simulink library "Kitchen_Lib"  (R2023a)
settings: Solver=VariableStepAuto  StartTime=0.0  StopTime=10.0  RelTol=1e-3  EnableMultiTasking=on
undefined symbols (not defined in the file): Kitc_BusTyp_P, Kitc_BusTypSkyr_C, Kitc_ColrLedColrls_C, Kitc_ColrLedGrn_C, Kitc_ColrLedRed_C, Kitc_ColrLedYlw_C, Kitc_StDgnWtrTank_C, Kitc_StElecPlugScktOffByClmp50_P, Kitc_StsDlyBlink_C, Kitc_StsErrBlink_C, Kitc_StsFctAcvn_P, Kitc_StsInfoBlink_C, Kitc_StsKitchnOffAutoIgOff_P, Kitc_StsKitchnOffBySwt_P, Kitc_StsKitchnOffDoorLockd_P, Kitc_StsKitchnOffIgOff_P, Kitc_StsKitchnOffUv_P, Kitc_StsKitchnOnBySwt_P, Kitc_StsKitchnOnNVM_P, Kitc_StsLedOff_C, Kitc_StsLedOn_C, Kitc_StsLrgCnsAcv_P, Kitc_StTrfrAnSwtInstd_P, Kitc_StTrfrSwtInstd_P, Kitc_TiKitcRefgtrOffDly_P, Kitc_ULowrThdBat_C, Kitc_UUpprThdBat_C, Kitc_ValFalse_C, Kitc_ValPwmFreq2_C, Kitc_ValPwmFreq_C, Kitc_ValTrue_C
libraries: MAN_Library x50, E2E_Lib x3
(part 12 of 13)

== system Kitchen_Lib/Kitchen/100ms/Kitchn/Subsystem1/Subsystem19/KSW_Battery/BatteryVoltageUnder23V/TurnOffDelay/TurnOffDelayOriginal/TimePulseOriginal/TimerCountingUpOriginal ==
  TimerEnable : Inport
  TimerReset : Inport  Port=2
  TimerThreshold : Inport  Port=3
  CycleTime : Inport  Port=4
  Data Type Conversion2 : DataTypeConversion  OutDataTypeStr=boolean  SaturateOnIntegerOverflow=off  RndMeth=Floor
  Data Type Conversion4 : DataTypeConversion  OutDataTypeStr=uint32  SaturateOnIntegerOverflow=off  RndMeth=Floor
  Data Type Conversion5 : DataTypeConversion  OutDataTypeStr=uint32  SaturateOnIntegerOverflow=off  RndMeth=Floor
  Data Type Conversion6 : DataTypeConversion  OutDataTypeStr=uint32  SaturateOnIntegerOverflow=off  RndMeth=Floor
  Data Type Conversion7 : DataTypeConversion  OutDataTypeStr=boolean  SaturateOnIntegerOverflow=off  RndMeth=Floor
  Delay : Delay  DelayLength=1  InitialCondition=0  ExternalReset=Rising
      settings: InputPortMap=u0,r5
  Delay1 : Delay  DelayLength=1  InitialCondition=0
  Logical Operator1 : Logic  Operator=NOT  AllPortsSameDT=off  OutDataTypeStr=boolean
  Logical Operator2 : Logic  AllPortsSameDT=off  OutDataTypeStr=boolean
  Logical Operator3 : Logic  Operator=OR  AllPortsSameDT=off  OutDataTypeStr=boolean
  Multiport Switch : MultiPortSwitch  DataPortOrder=Zero-based contiguous  Inputs=2  zeroidx=on  SaturateOnIntegerOverflow=off  InputSameDT=off
  Multiport Switch1 : MultiPortSwitch  DataPortOrder=Zero-based contiguous  Inputs=2  zeroidx=on  SaturateOnIntegerOverflow=off  InputSameDT=off
  Multiport Switch2 : MultiPortSwitch  DataPortOrder=Zero-based contiguous  Inputs=2  zeroidx=on  SaturateOnIntegerOverflow=off  InputSameDT=off
  Relational Operator : RelationalOperator  OutDataTypeStr=boolean  InputSameDT=off
  Relational Operator1 : RelationalOperator  Operator===  OutDataTypeStr=boolean  InputSameDT=off
  RisingEdgeDetection : Subsystem  AncestorBlock=MAN_Library/RisingEdgeDetection
  StartValue_ms1 : Constant  Value=uint32(4294967295)  OutDataTypeStr=uint32
  StartValue_ms2 : Constant  Value=uint32(4294967295)  OutDataTypeStr=uint32
  StartValue_ms3 : Constant  Value=uint32(0)  OutDataTypeStr=uint32
  StartValue_ms5 : Constant  Value=uint32(4294967295)  OutDataTypeStr=uint32
  Sum : Sum
  U32_Saturation : Subsystem  AncestorBlock=MAN_Library/U32_Saturation
  TimerFlag : Outport
  TimerCurrentValue : Outport  Port=2
  wires:
  CycleTime/1 -> Data Type Conversion4/1
  Data Type Conversion2/1 -> Logical Operator3/1
  RisingEdgeDetection/1(Q) -> Logical Operator3/2
  TimerReset/1 -> Data Type Conversion2/1
  TimerEnable/1 -> Data Type Conversion7/1
  Data Type Conversion6/1 -> Relational Operator/2
  Data Type Conversion4/1 -> Sum/2
  StartValue_ms3/1 -> U32_Saturation/3(LowerLimit), Multiport Switch/3
  Multiport Switch2/1 -> U32_Saturation/2(IN)
  Sum/1 -> Multiport Switch2/2
  StartValue_ms2/1 -> Multiport Switch2/3
  Relational Operator1/1 -> Multiport Switch2/1
  Delay/1 -> Multiport Switch1/2, Relational Operator1/1, Sum/1
  StartValue_ms5/1 -> Relational Operator1/2
  Logical Operator3/1 -> Multiport Switch/1, [ResetTimer_BOOL]
  StartValue_ms1/1 -> U32_Saturation/1(UpperLimit)
  Delay1/1 -> Logical Operator1/1
  U32_Saturation/1(OUT) -> Multiport Switch1/3
  Logical Operator1/1 -> Logical Operator2/2
  Logical Operator2/1 -> Multiport Switch1/1
  Data Type Conversion5/1 -> TimerCurrentValue/1, Delay/1, Relational Operator/1
  Data Type Conversion7/1 -> Logical Operator2/1, RisingEdgeDetection/1(CLK)
  Multiport Switch/1 -> Data Type Conversion5/1
  Relational Operator/1 -> TimerFlag/1, Delay1/1
  Multiport Switch1/1 -> Multiport Switch/2
  TimerThreshold/1 -> Data Type Conversion6/1
  [ResetTimer_BOOL] -> Delay/2

== system Kitchen_Lib/Kitchen/100ms/Kitchn/Subsystem1/Subsystem19/KitchenEnable/KitchenOffAutomaticIgnitionOff/TurnOnDelay/TurnOnDelayOriginal/TimePulseOriginal/RisingEdgeDetection ==
  CLK : Inport
  Constant : Constant  Value=boolean(1)  OutDataTypeStr=boolean
  Data Type Conversion1 : DataTypeConversion  OutDataTypeStr=boolean  SaturateOnIntegerOverflow=off  RndMeth=Floor
  Logical Operator : Logic  AllPortsSameDT=off  OutDataTypeStr=boolean
  Relational Operator : RelationalOperator  Operator=~=  OutDataTypeStr=boolean  InputSameDT=off
  Relational Operator1 : RelationalOperator  Operator===  OutDataTypeStr=boolean  InputSameDT=off
  Unit Delay : UnitDelay  SampleTime=-1  HasFrameUpgradeWarning=on
  Q : Outport
  wires:
  Data Type Conversion1/1 -> Relational Operator1/1, Relational Operator/2, Unit Delay/1
  Constant/1 -> Relational Operator1/2
  Logical Operator/1 -> Q/1
  Relational Operator1/1 -> Logical Operator/2
  Relational Operator/1 -> Logical Operator/1
  Unit Delay/1 -> Relational Operator/1
  CLK/1 -> Data Type Conversion1/1

== system Kitchen_Lib/Kitchen/100ms/Kitchn/Subsystem1/Subsystem19/KitchenEnable/KitchenOffAutomaticIgnitionOff/TurnOnDelay/TurnOnDelayOriginal/TimePulseOriginal/RisingEdgeDetection1 ==
  CLK : Inport
  Constant : Constant  Value=boolean(1)  OutDataTypeStr=boolean
  Data Type Conversion1 : DataTypeConversion  OutDataTypeStr=boolean  SaturateOnIntegerOverflow=off  RndMeth=Floor
  Logical Operator : Logic  AllPortsSameDT=off  OutDataTypeStr=boolean
  Relational Operator : RelationalOperator  Operator=~=  OutDataTypeStr=boolean  InputSameDT=off
  Relational Operator1 : RelationalOperator  Operator===  OutDataTypeStr=boolean  InputSameDT=off
  Unit Delay : UnitDelay  SampleTime=-1  HasFrameUpgradeWarning=on
  Q : Outport
  wires:
  Data Type Conversion1/1 -> Relational Operator1/1, Relational Operator/2, Unit Delay/1
  Constant/1 -> Relational Operator1/2
  Logical Operator/1 -> Q/1
  Relational Operator1/1 -> Logical Operator/2
  Relational Operator/1 -> Logical Operator/1
  Unit Delay/1 -> Relational Operator/1
  CLK/1 -> Data Type Conversion1/1

== system Kitchen_Lib/Kitchen/100ms/Kitchn/Subsystem1/Subsystem19/KitchenEnable/KitchenOffAutomaticIgnitionOff/TurnOnDelay/TurnOnDelayOriginal/TimePulseOriginal/SR ==
  S : Inport
  R : Inport  Port=2
  Constant1 : Constant  Value=boolean(1)  OutDataTypeStr=boolean
  Constant3 : Constant  Value=boolean(0)  OutDataTypeStr=boolean
  Data Type Conversion1 : DataTypeConversion  OutDataTypeStr=boolean  SaturateOnIntegerOverflow=off  RndMeth=Floor
  Data Type Conversion2 : DataTypeConversion  OutDataTypeStr=boolean  SaturateOnIntegerOverflow=off  RndMeth=Floor
  Multiport Switch : MultiPortSwitch  DataPortOrder=Zero-based contiguous  Inputs=2  zeroidx=on  SaturateOnIntegerOverflow=off  InputSameDT=off
  Multiport Switch1 : MultiPortSwitch  DataPortOrder=Zero-based contiguous  Inputs=2  zeroidx=on  SaturateOnIntegerOverflow=off  InputSameDT=off
  Unit Delay : UnitDelay  SampleTime=-1  HasFrameUpgradeWarning=on
  Q : Outport
  wires:
  Data Type Conversion2/1 -> Multiport Switch/1
  Data Type Conversion1/1 -> Multiport Switch1/1
  Constant3/1 -> Multiport Switch1/3
  Multiport Switch/1 -> Unit Delay/1, Q/1
  Unit Delay/1 -> Multiport Switch1/2
  R/1 -> Data Type Conversion1/1
  Multiport Switch1/1 -> Multiport Switch/2
  Constant1/1 -> Multiport Switch/3
  S/1 -> Data Type Conversion2/1

== system Kitchen_Lib/Kitchen/100ms/Kitchn/Subsystem1/Subsystem19/KitchenEnable/KitchenOffAutomaticIgnitionOff/TurnOnDelay/TurnOnDelayOriginal/TimePulseOriginal/TimerCountingUpOriginal ==
  TimerEnable : Inport
  TimerReset : Inport  Port=2
  TimerThreshold : Inport  Port=3
  CycleTime : Inport  Port=4
  Data Type Conversion2 : DataTypeConversion  OutDataTypeStr=boolean  SaturateOnIntegerOverflow=off  RndMeth=Floor
  Data Type Conversion4 : DataTypeConversion  OutDataTypeStr=uint32  SaturateOnIntegerOverflow=off  RndMeth=Floor
  Data Type Conversion5 : DataTypeConversion  OutDataTypeStr=uint32  SaturateOnIntegerOverflow=off  RndMeth=Floor
  Data Type Conversion6 : DataTypeConversion  OutDataTypeStr=uint32  SaturateOnIntegerOverflow=off  RndMeth=Floor
  Data Type Conversion7 : DataTypeConversion  OutDataTypeStr=boolean  SaturateOnIntegerOverflow=off  RndMeth=Floor
  Delay : Delay  DelayLength=1  InitialCondition=0  ExternalReset=Rising
      settings: InputPortMap=u0,r5
  Delay1 : Delay  DelayLength=1  InitialCondition=0
  Logical Operator1 : Logic  Operator=NOT  AllPortsSameDT=off  OutDataTypeStr=boolean
  Logical Operator2 : Logic  AllPortsSameDT=off  OutDataTypeStr=boolean
  Logical Operator3 : Logic  Operator=OR  AllPortsSameDT=off  OutDataTypeStr=boolean
  Multiport Switch : MultiPortSwitch  DataPortOrder=Zero-based contiguous  Inputs=2  zeroidx=on  SaturateOnIntegerOverflow=off  InputSameDT=off
  Multiport Switch1 : MultiPortSwitch  DataPortOrder=Zero-based contiguous  Inputs=2  zeroidx=on  SaturateOnIntegerOverflow=off  InputSameDT=off
  Multiport Switch2 : MultiPortSwitch  DataPortOrder=Zero-based contiguous  Inputs=2  zeroidx=on  SaturateOnIntegerOverflow=off  InputSameDT=off
  Relational Operator : RelationalOperator  OutDataTypeStr=boolean  InputSameDT=off
  Relational Operator1 : RelationalOperator  Operator===  OutDataTypeStr=boolean  InputSameDT=off
  RisingEdgeDetection : Subsystem  AncestorBlock=MAN_Library/RisingEdgeDetection
  StartValue_ms1 : Constant  Value=uint32(4294967295)  OutDataTypeStr=uint32
  StartValue_ms2 : Constant  Value=uint32(4294967295)  OutDataTypeStr=uint32
  StartValue_ms3 : Constant  Value=uint32(0)  OutDataTypeStr=uint32
  StartValue_ms5 : Constant  Value=uint32(4294967295)  OutDataTypeStr=uint32
  Sum : Sum
  U32_Saturation : Subsystem  AncestorBlock=MAN_Library/U32_Saturation
  TimerFlag : Outport
  TimerCurrentValue : Outport  Port=2
  wires:
  CycleTime/1 -> Data Type Conversion4/1
  Data Type Conversion2/1 -> Logical Operator3/1
  RisingEdgeDetection/1(Q) -> Logical Operator3/2
  TimerReset/1 -> Data Type Conversion2/1
  TimerEnable/1 -> Data Type Conversion7/1
  Data Type Conversion6/1 -> Relational Operator/2
  Data Type Conversion4/1 -> Sum/2
  StartValue_ms3/1 -> U32_Saturation/3(LowerLimit), Multiport Switch/3
  Multiport Switch2/1 -> U32_Saturation/2(IN)
  Sum/1 -> Multiport Switch2/2
  StartValue_ms2/1 -> Multiport Switch2/3
  Relational Operator1/1 -> Multiport Switch2/1
  Delay/1 -> Multiport Switch1/2, Relational Operator1/1, Sum/1
  StartValue_ms5/1 -> Relational Operator1/2
  Logical Operator3/1 -> Multiport Switch/1, [ResetTimer_BOOL]
  StartValue_ms1/1 -> U32_Saturation/1(UpperLimit)
  Delay1/1 -> Logical Operator1/1
  U32_Saturation/1(OUT) -> Multiport Switch1/3
  Logical Operator1/1 -> Logical Operator2/2
  Logical Operator2/1 -> Multiport Switch1/1
  Data Type Conversion5/1 -> TimerCurrentValue/1, Delay/1, Relational Operator/1
  Data Type Conversion7/1 -> Logical Operator2/1, RisingEdgeDetection/1(CLK)
  Multiport Switch/1 -> Data Type Conversion5/1
  Relational Operator/1 -> TimerFlag/1, Delay1/1
  Multiport Switch1/1 -> Multiport Switch/2
  TimerThreshold/1 -> Data Type Conversion6/1
  [ResetTimer_BOOL] -> Delay/2

== system Kitchen_Lib/Kitchen/100ms/Kitchn/Subsystem1/Subsystem19/KitchenEnable/Subsystem/TurnOnDelay/TurnOnDelayOriginal/TimePulseOriginal/RisingEdgeDetection ==
  CLK : Inport
  Constant : Constant  Value=boolean(1)  OutDataTypeStr=boolean
  Data Type Conversion1 : DataTypeConversion  OutDataTypeStr=boolean  SaturateOnIntegerOverflow=off  RndMeth=Floor
  Logical Operator : Logic  AllPortsSameDT=off  OutDataTypeStr=boolean
  Relational Operator : RelationalOperator  Operator=~=  OutDataTypeStr=boolean  InputSameDT=off
  Relational Operator1 : RelationalOperator  Operator===  OutDataTypeStr=boolean  InputSameDT=off
  Unit Delay : UnitDelay  SampleTime=-1  HasFrameUpgradeWarning=on
  Q : Outport
  wires:
  Data Type Conversion1/1 -> Relational Operator1/1, Relational Operator/2, Unit Delay/1
  Constant/1 -> Relational Operator1/2
  Logical Operator/1 -> Q/1
  Relational Operator1/1 -> Logical Operator/2
  Relational Operator/1 -> Logical Operator/1
  Unit Delay/1 -> Relational Operator/1
  CLK/1 -> Data Type Conversion1/1

== system Kitchen_Lib/Kitchen/100ms/Kitchn/Subsystem1/Subsystem19/KitchenEnable/Subsystem/TurnOnDelay/TurnOnDelayOriginal/TimePulseOriginal/RisingEdgeDetection1 ==
  CLK : Inport
  Constant : Constant  Value=boolean(1)  OutDataTypeStr=boolean
  Data Type Conversion1 : DataTypeConversion  OutDataTypeStr=boolean  SaturateOnIntegerOverflow=off  RndMeth=Floor
  Logical Operator : Logic  AllPortsSameDT=off  OutDataTypeStr=boolean
  Relational Operator : RelationalOperator  Operator=~=  OutDataTypeStr=boolean  InputSameDT=off
  Relational Operator1 : RelationalOperator  Operator===  OutDataTypeStr=boolean  InputSameDT=off
  Unit Delay : UnitDelay  SampleTime=-1  HasFrameUpgradeWarning=on
  Q : Outport
  wires:
  Data Type Conversion1/1 -> Relational Operator1/1, Relational Operator/2, Unit Delay/1
  Constant/1 -> Relational Operator1/2
  Logical Operator/1 -> Q/1
  Relational Operator1/1 -> Logical Operator/2
  Relational Operator/1 -> Logical Operator/1
  Unit Delay/1 -> Relational Operator/1
  CLK/1 -> Data Type Conversion1/1

== system Kitchen_Lib/Kitchen/100ms/Kitchn/Subsystem1/Subsystem19/KitchenEnable/Subsystem/TurnOnDelay/TurnOnDelayOriginal/TimePulseOriginal/SR ==
  S : Inport
  R : Inport  Port=2
  Constant1 : Constant  Value=boolean(1)  OutDataTypeStr=boolean
  Constant3 : Constant  Value=boolean(0)  OutDataTypeStr=boolean
  Data Type Conversion1 : DataTypeConversion  OutDataTypeStr=boolean  SaturateOnIntegerOverflow=off  RndMeth=Floor
  Data Type Conversion2 : DataTypeConversion  OutDataTypeStr=boolean  SaturateOnIntegerOverflow=off  RndMeth=Floor
  Multiport Switch : MultiPortSwitch  DataPortOrder=Zero-based contiguous  Inputs=2  zeroidx=on  SaturateOnIntegerOverflow=off  InputSameDT=off
  Multiport Switch1 : MultiPortSwitch  DataPortOrder=Zero-based contiguous  Inputs=2  zeroidx=on  SaturateOnIntegerOverflow=off  InputSameDT=off
  Unit Delay : UnitDelay  SampleTime=-1  HasFrameUpgradeWarning=on
  Q : Outport
  wires:
  Data Type Conversion2/1 -> Multiport Switch/1
  Data Type Conversion1/1 -> Multiport Switch1/1
  Constant3/1 -> Multiport Switch1/3
  Multiport Switch/1 -> Unit Delay/1, Q/1
  Unit Delay/1 -> Multiport Switch1/2
  R/1 -> Data Type Conversion1/1
  Multiport Switch1/1 -> Multiport Switch/2
  Constant1/1 -> Multiport Switch/3
  S/1 -> Data Type Conversion2/1

== system Kitchen_Lib/Kitchen/100ms/Kitchn/Subsystem1/Subsystem19/KitchenEnable/Subsystem/TurnOnDelay/TurnOnDelayOriginal/TimePulseOriginal/TimerCountingUpOriginal ==
  TimerEnable : Inport
  TimerReset : Inport  Port=2
  TimerThreshold : Inport  Port=3
  CycleTime : Inport  Port=4
  Data Type Conversion2 : DataTypeConversion  OutDataTypeStr=boolean  SaturateOnIntegerOverflow=off  RndMeth=Floor
  Data Type Conversion4 : DataTypeConversion  OutDataTypeStr=uint32  SaturateOnIntegerOverflow=off  RndMeth=Floor
  Data Type Conversion5 : DataTypeConversion  OutDataTypeStr=uint32  SaturateOnIntegerOverflow=off  RndMeth=Floor
  Data Type Conversion6 : DataTypeConversion  OutDataTypeStr=uint32  SaturateOnIntegerOverflow=off  RndMeth=Floor
  Data Type Conversion7 : DataTypeConversion  OutDataTypeStr=boolean  SaturateOnIntegerOverflow=off  RndMeth=Floor
  Delay : Delay  DelayLength=1  InitialCondition=0  ExternalReset=Rising
      settings: InputPortMap=u0,r5
  Delay1 : Delay  DelayLength=1  InitialCondition=0
  Logical Operator1 : Logic  Operator=NOT  AllPortsSameDT=off  OutDataTypeStr=boolean
  Logical Operator2 : Logic  AllPortsSameDT=off  OutDataTypeStr=boolean
  Logical Operator3 : Logic  Operator=OR  AllPortsSameDT=off  OutDataTypeStr=boolean
  Multiport Switch : MultiPortSwitch  DataPortOrder=Zero-based contiguous  Inputs=2  zeroidx=on  SaturateOnIntegerOverflow=off  InputSameDT=off
  Multiport Switch1 : MultiPortSwitch  DataPortOrder=Zero-based contiguous  Inputs=2  zeroidx=on  SaturateOnIntegerOverflow=off  InputSameDT=off
  Multiport Switch2 : MultiPortSwitch  DataPortOrder=Zero-based contiguous  Inputs=2  zeroidx=on  SaturateOnIntegerOverflow=off  InputSameDT=off
  Relational Operator : RelationalOperator  OutDataTypeStr=boolean  InputSameDT=off
  Relational Operator1 : RelationalOperator  Operator===  OutDataTypeStr=boolean  InputSameDT=off
  RisingEdgeDetection : Subsystem  AncestorBlock=MAN_Library/RisingEdgeDetection
  StartValue_ms1 : Constant  Value=uint32(4294967295)  OutDataTypeStr=uint32
  StartValue_ms2 : Constant  Value=uint32(4294967295)  OutDataTypeStr=uint32
  StartValue_ms3 : Constant  Value=uint32(0)  OutDataTypeStr=uint32
  StartValue_ms5 : Constant  Value=uint32(4294967295)  OutDataTypeStr=uint32
  Sum : Sum
  U32_Saturation : Subsystem  AncestorBlock=MAN_Library/U32_Saturation
  TimerFlag : Outport
  TimerCurrentValue : Outport  Port=2
  wires:
  CycleTime/1 -> Data Type Conversion4/1
  Data Type Conversion2/1 -> Logical Operator3/1
  RisingEdgeDetection/1(Q) -> Logical Operator3/2
  TimerReset/1 -> Data Type Conversion2/1
  TimerEnable/1 -> Data Type Conversion7/1
  Data Type Conversion6/1 -> Relational Operator/2
  Data Type Conversion4/1 -> Sum/2
  StartValue_ms3/1 -> U32_Saturation/3(LowerLimit), Multiport Switch/3
  Multiport Switch2/1 -> U32_Saturation/2(IN)
  Sum/1 -> Multiport Switch2/2
  StartValue_ms2/1 -> Multiport Switch2/3
  Relational Operator1/1 -> Multiport Switch2/1
  Delay/1 -> Multiport Switch1/2, Relational Operator1/1, Sum/1
  StartValue_ms5/1 -> Relational Operator1/2
  Logical Operator3/1 -> Multiport Switch/1, [ResetTimer_BOOL]
  StartValue_ms1/1 -> U32_Saturation/1(UpperLimit)
  Delay1/1 -> Logical Operator1/1
  U32_Saturation/1(OUT) -> Multiport Switch1/3
  Logical Operator1/1 -> Logical Operator2/2
  Logical Operator2/1 -> Multiport Switch1/1
  Data Type Conversion5/1 -> TimerCurrentValue/1, Delay/1, Relational Operator/1
  Data Type Conversion7/1 -> Logical Operator2/1, RisingEdgeDetection/1(CLK)
  Multiport Switch/1 -> Data Type Conversion5/1
  Relational Operator/1 -> TimerFlag/1, Delay1/1
  Multiport Switch1/1 -> Multiport Switch/2
  TimerThreshold/1 -> Data Type Conversion6/1
  [ResetTimer_BOOL] -> Delay/2

== system Kitchen_Lib/Kitchen/100ms/Kitchn/Subsystem1/Subsystem19/KitchenSwtLed/KitchenError/TurnOffDelay/TurnOffDelayOriginal/TimePulseOriginal/RisingEdgeDetection ==
  CLK : Inport
  Constant : Constant  Value=boolean(1)  OutDataTypeStr=boolean
  Data Type Conversion1 : DataTypeConversion  OutDataTypeStr=boolean  SaturateOnIntegerOverflow=off  RndMeth=Floor
  Logical Operator : Logic  AllPortsSameDT=off  OutDataTypeStr=boolean
  Relational Operator : RelationalOperator  Operator=~=  OutDataTypeStr=boolean  InputSameDT=off
  Relational Operator1 : RelationalOperator  Operator===  OutDataTypeStr=boolean  InputSameDT=off
  Unit Delay : UnitDelay  SampleTime=-1  HasFrameUpgradeWarning=on
  Q : Outport
  wires:
  Data Type Conversion1/1 -> Relational Operator1/1, Relational Operator/2, Unit Delay/1
  Constant/1 -> Relational Operator1/2
  Logical Operator/1 -> Q/1
  Relational Operator1/1 -> Logical Operator/2
  Relational Operator/1 -> Logical Operator/1
  Unit Delay/1 -> Relational Operator/1
  CLK/1 -> Data Type Conversion1/1

== system Kitchen_Lib/Kitchen/100ms/Kitchn/Subsystem1/Subsystem19/KitchenSwtLed/KitchenError/TurnOffDelay/TurnOffDelayOriginal/TimePulseOriginal/RisingEdgeDetection1 ==
  CLK : Inport
  Constant : Constant  Value=boolean(1)  OutDataTypeStr=boolean
  Data Type Conversion1 : DataTypeConversion  OutDataTypeStr=boolean  SaturateOnIntegerOverflow=off  RndMeth=Floor
  Logical Operator : Logic  AllPortsSameDT=off  OutDataTypeStr=boolean
  Relational Operator : RelationalOperator  Operator=~=  OutDataTypeStr=boolean  InputSameDT=off
  Relational Operator1 : RelationalOperator  Operator===  OutDataTypeStr=boolean  InputSameDT=off
  Unit Delay : UnitDelay  SampleTime=-1  HasFrameUpgradeWarning=on
  Q : Outport
  wires:
  Data Type Conversion1/1 -> Relational Operator1/1, Relational Operator/2, Unit Delay/1
  Constant/1 -> Relational Operator1/2
  Logical Operator/1 -> Q/1
  Relational Operator1/1 -> Logical Operator/2
  Relational Operator/1 -> Logical Operator/1
  Unit Delay/1 -> Relational Operator/1
  CLK/1 -> Data Type Conversion1/1

== system Kitchen_Lib/Kitchen/100ms/Kitchn/Subsystem1/Subsystem19/KitchenSwtLed/KitchenError/TurnOffDelay/TurnOffDelayOriginal/TimePulseOriginal/SR ==
  S : Inport
  R : Inport  Port=2
  Constant1 : Constant  Value=boolean(1)  OutDataTypeStr=boolean
  Constant3 : Constant  Value=boolean(0)  OutDataTypeStr=boolean
  Data Type Conversion1 : DataTypeConversion  OutDataTypeStr=boolean  SaturateOnIntegerOverflow=off  RndMeth=Floor
  Data Type Conversion2 : DataTypeConversion  OutDataTypeStr=boolean  SaturateOnIntegerOverflow=off  RndMeth=Floor
  Multiport Switch : MultiPortSwitch  DataPortOrder=Zero-based contiguous  Inputs=2  zeroidx=on  SaturateOnIntegerOverflow=off  InputSameDT=off
  Multiport Switch1 : MultiPortSwitch  DataPortOrder=Zero-based contiguous  Inputs=2  zeroidx=on  SaturateOnIntegerOverflow=off  InputSameDT=off
  Unit Delay : UnitDelay  SampleTime=-1  HasFrameUpgradeWarning=on
  Q : Outport
  wires:
  Data Type Conversion2/1 -> Multiport Switch/1
  Data Type Conversion1/1 -> Multiport Switch1/1
  Constant3/1 -> Multiport Switch1/3
  Multiport Switch/1 -> Unit Delay/1, Q/1
  Unit Delay/1 -> Multiport Switch1/2
  R/1 -> Data Type Conversion1/1
  Multiport Switch1/1 -> Multiport Switch/2
  Constant1/1 -> Multiport Switch/3
  S/1 -> Data Type Conversion2/1

== system Kitchen_Lib/Kitchen/100ms/Kitchn/Subsystem1/Subsystem19/KitchenSwtLed/KitchenError/TurnOffDelay/TurnOffDelayOriginal/TimePulseOriginal/TimerCountingUpOriginal ==
  TimerEnable : Inport
  TimerReset : Inport  Port=2
  TimerThreshold : Inport  Port=3
  CycleTime : Inport  Port=4
  Data Type Conversion2 : DataTypeConversion  OutDataTypeStr=boolean  SaturateOnIntegerOverflow=off  RndMeth=Floor
  Data Type Conversion4 : DataTypeConversion  OutDataTypeStr=uint32  SaturateOnIntegerOverflow=off  RndMeth=Floor
  Data Type Conversion5 : DataTypeConversion  OutDataTypeStr=uint32  SaturateOnIntegerOverflow=off  RndMeth=Floor
  Data Type Conversion6 : DataTypeConversion  OutDataTypeStr=uint32  SaturateOnIntegerOverflow=off  RndMeth=Floor
  Data Type Conversion7 : DataTypeConversion  OutDataTypeStr=boolean  SaturateOnIntegerOverflow=off  RndMeth=Floor
  Delay : Delay  DelayLength=1  InitialCondition=0  ExternalReset=Rising
      settings: InputPortMap=u0,r5
  Delay1 : Delay  DelayLength=1  InitialCondition=0
  Logical Operator1 : Logic  Operator=NOT  AllPortsSameDT=off  OutDataTypeStr=boolean
  Logical Operator2 : Logic  AllPortsSameDT=off  OutDataTypeStr=boolean
  Logical Operator3 : Logic  Operator=OR  AllPortsSameDT=off  OutDataTypeStr=boolean
  Multiport Switch : MultiPortSwitch  DataPortOrder=Zero-based contiguous  Inputs=2  zeroidx=on  SaturateOnIntegerOverflow=off  InputSameDT=off
  Multiport Switch1 : MultiPortSwitch  DataPortOrder=Zero-based contiguous  Inputs=2  zeroidx=on  SaturateOnIntegerOverflow=off  InputSameDT=off
  Multiport Switch2 : MultiPortSwitch  DataPortOrder=Zero-based contiguous  Inputs=2  zeroidx=on  SaturateOnIntegerOverflow=off  InputSameDT=off
  Relational Operator : RelationalOperator  OutDataTypeStr=boolean  InputSameDT=off
  Relational Operator1 : RelationalOperator  Operator===  OutDataTypeStr=boolean  InputSameDT=off
  RisingEdgeDetection : Subsystem  AncestorBlock=MAN_Library/RisingEdgeDetection
  StartValue_ms1 : Constant  Value=uint32(4294967295)  OutDataTypeStr=uint32
  StartValue_ms2 : Constant  Value=uint32(4294967295)  OutDataTypeStr=uint32
  StartValue_ms3 : Constant  Value=uint32(0)  OutDataTypeStr=uint32
  StartValue_ms5 : Constant  Value=uint32(4294967295)  OutDataTypeStr=uint32
  Sum : Sum
  U32_Saturation : Subsystem  AncestorBlock=MAN_Library/U32_Saturation
  TimerFlag : Outport
  TimerCurrentValue : Outport  Port=2
  wires:
  CycleTime/1 -> Data Type Conversion4/1
  Data Type Conversion2/1 -> Logical Operator3/1
  RisingEdgeDetection/1(Q) -> Logical Operator3/2
  TimerReset/1 -> Data Type Conversion2/1
  TimerEnable/1 -> Data Type Conversion7/1
  Data Type Conversion6/1 -> Relational Operator/2
  Data Type Conversion4/1 -> Sum/2
  StartValue_ms3/1 -> U32_Saturation/3(LowerLimit), Multiport Switch/3
  Multiport Switch2/1 -> U32_Saturation/2(IN)
  Sum/1 -> Multiport Switch2/2
  StartValue_ms2/1 -> Multiport Switch2/3
  Relational Operator1/1 -> Multiport Switch2/1
  Delay/1 -> Multiport Switch1/2, Relational Operator1/1, Sum/1
  StartValue_ms5/1 -> Relational Operator1/2
  Logical Operator3/1 -> Multiport Switch/1, [ResetTimer_BOOL]
  StartValue_ms1/1 -> U32_Saturation/1(UpperLimit)
  Delay1/1 -> Logical Operator1/1
  U32_Saturation/1(OUT) -> Multiport Switch1/3
  Logical Operator1/1 -> Logical Operator2/2
  Logical Operator2/1 -> Multiport Switch1/1
  Data Type Conversion5/1 -> TimerCurrentValue/1, Delay/1, Relational Operator/1
  Data Type Conversion7/1 -> Logical Operator2/1, RisingEdgeDetection/1(CLK)
  Multiport Switch/1 -> Data Type Conversion5/1
  Relational Operator/1 -> TimerFlag/1, Delay1/1
  Multiport Switch1/1 -> Multiport Switch/2
  TimerThreshold/1 -> Data Type Conversion6/1
  [ResetTimer_BOOL] -> Delay/2

== system Kitchen_Lib/Kitchen/100ms/Kitchn/Subsystem1/Subsystem19/KitchenSwtLed/TurnOffDelay1/TurnOffDelayOriginal/TimePulseOriginal/TimerCountingUpOriginal/RisingEdgeDetection ==
  CLK : Inport
  Constant : Constant  Value=boolean(1)  OutDataTypeStr=boolean
  Data Type Conversion1 : DataTypeConversion  OutDataTypeStr=boolean  SaturateOnIntegerOverflow=off  RndMeth=Floor
  Logical Operator : Logic  AllPortsSameDT=off  OutDataTypeStr=boolean
  Relational Operator : RelationalOperator  Operator=~=  OutDataTypeStr=boolean  InputSameDT=off
  Relational Operator1 : RelationalOperator  Operator===  OutDataTypeStr=boolean  InputSameDT=off
  Unit Delay : UnitDelay  SampleTime=-1  HasFrameUpgradeWarning=on
  Q : Outport
  wires:
  Data Type Conversion1/1 -> Relational Operator1/1, Relational Operator/2, Unit Delay/1
  Constant/1 -> Relational Operator1/2
  Logical Operator/1 -> Q/1
  Relational Operator1/1 -> Logical Operator/2
  Relational Operator/1 -> Logical Operator/1
  Unit Delay/1 -> Relational Operator/1
  CLK/1 -> Data Type Conversion1/1

== system Kitchen_Lib/Kitchen/100ms/Kitchn/Subsystem1/Subsystem19/KitchenSwtLed/TurnOffDelay1/TurnOffDelayOriginal/TimePulseOriginal/TimerCountingUpOriginal/U32_Saturation ==
  UpperLimit : Inport
  IN : Inport  Port=2
  LowerLimit : Inport  Port=3
  Data Type Conversion{1..4} (4 alike) : DataTypeConversion  OutDataTypeStr=uint32  SaturateOnIntegerOverflow=off  RndMeth=Floor
  MinMax : MinMax  Inputs=2  OutDataTypeStr=uint32
  MinMax1 : MinMax  Function=max  Inputs=2  OutDataTypeStr=uint32
  OUT : Outport
  wires:
  Data Type Conversion3/1 -> OUT/1
  Data Type Conversion2/1 -> MinMax/1
  Data Type Conversion1/1 -> MinMax/2
  Data Type Conversion4/1 -> MinMax1/1
  MinMax1/1 -> Data Type Conversion3/1
  LowerLimit/1 -> Data Type Conversion4/1
  MinMax/1 -> MinMax1/2
  IN/1 -> Data Type Conversion2/1
  UpperLimit/1 -> Data Type Conversion1/1

== system Kitchen_Lib/Kitchen/100ms/Kitchn/Subsystem1/Subsystem19/Refgtr/TurnOffDelay/TurnOffDelayOriginal/TimePulseOriginal/TimerCountingUpOriginal/RisingEdgeDetection ==
  CLK : Inport
  Constant : Constant  Value=boolean(1)  OutDataTypeStr=boolean
  Data Type Conversion1 : DataTypeConversion  OutDataTypeStr=boolean  SaturateOnIntegerOverflow=off  RndMeth=Floor
  Logical Operator : Logic  AllPortsSameDT=off  OutDataTypeStr=boolean
  Relational Operator : RelationalOperator  Operator=~=  OutDataTypeStr=boolean  InputSameDT=off
  Relational Operator1 : RelationalOperator  Operator===  OutDataTypeStr=boolean  InputSameDT=off
  Unit Delay : UnitDelay  SampleTime=-1  HasFrameUpgradeWarning=on
  Q : Outport
  wires:
  Data Type Conversion1/1 -> Relational Operator1/1, Relational Operator/2, Unit Delay/1
  Constant/1 -> Relational Operator1/2
  Logical Operator/1 -> Q/1
  Relational Operator1/1 -> Logical Operator/2
  Relational Operator/1 -> Logical Operator/1
  Unit Delay/1 -> Relational Operator/1
  CLK/1 -> Data Type Conversion1/1

== system Kitchen_Lib/Kitchen/100ms/Kitchn/Subsystem1/Subsystem19/Refgtr/TurnOffDelay/TurnOffDelayOriginal/TimePulseOriginal/TimerCountingUpOriginal/U32_Saturation ==
  UpperLimit : Inport
  IN : Inport  Port=2
  LowerLimit : Inport  Port=3
  Data Type Conversion{1..4} (4 alike) : DataTypeConversion  OutDataTypeStr=uint32  SaturateOnIntegerOverflow=off  RndMeth=Floor
  MinMax : MinMax  Inputs=2  OutDataTypeStr=uint32
  MinMax1 : MinMax  Function=max  Inputs=2  OutDataTypeStr=uint32
  OUT : Outport
  wires:
  Data Type Conversion3/1 -> OUT/1
  Data Type Conversion2/1 -> MinMax/1
  Data Type Conversion1/1 -> MinMax/2
  Data Type Conversion4/1 -> MinMax1/1
  MinMax1/1 -> Data Type Conversion3/1
  LowerLimit/1 -> Data Type Conversion4/1
  MinMax/1 -> MinMax1/2
  IN/1 -> Data Type Conversion2/1
  UpperLimit/1 -> Data Type Conversion1/1

== system Kitchen_Lib/Kitchen/100ms/Kitchn/Subsystem1/Subsystem19/Trfr/TurnOnDelay/TurnOnDelayOriginal/TimePulseOriginal/TimerCountingUpOriginal/RisingEdgeDetection ==
  CLK : Inport
  Constant : Constant  Value=boolean(1)  OutDataTypeStr=boolean
  Data Type Conversion1 : DataTypeConversion  OutDataTypeStr=boolean  SaturateOnIntegerOverflow=off  RndMeth=Floor
  Logical Operator : Logic  AllPortsSameDT=off  OutDataTypeStr=boolean
  Relational Operator : RelationalOperator  Operator=~=  OutDataTypeStr=boolean  InputSameDT=off
  Relational Operator1 : RelationalOperator  Operator===  OutDataTypeStr=boolean  InputSameDT=off
  Unit Delay : UnitDelay  SampleTime=-1  HasFrameUpgradeWarning=on
  Q : Outport
  wires:
  Data Type Conversion1/1 -> Relational Operator1/1, Relational Operator/2, Unit Delay/1
  Constant/1 -> Relational Operator1/2
  Logical Operator/1 -> Q/1
  Relational Operator1/1 -> Logical Operator/2
  Relational Operator/1 -> Logical Operator/1
  Unit Delay/1 -> Relational Operator/1
  CLK/1 -> Data Type Conversion1/1

== system Kitchen_Lib/Kitchen/100ms/Kitchn/Subsystem1/Subsystem19/Trfr/TurnOnDelay/TurnOnDelayOriginal/TimePulseOriginal/TimerCountingUpOriginal/U32_Saturation ==
  UpperLimit : Inport
  IN : Inport  Port=2
  LowerLimit : Inport  Port=3
  Data Type Conversion{1..4} (4 alike) : DataTypeConversion  OutDataTypeStr=uint32  SaturateOnIntegerOverflow=off  RndMeth=Floor
  MinMax : MinMax  Inputs=2  OutDataTypeStr=uint32
  MinMax1 : MinMax  Function=max  Inputs=2  OutDataTypeStr=uint32
  OUT : Outport
  wires:
  Data Type Conversion3/1 -> OUT/1
  Data Type Conversion2/1 -> MinMax/1
  Data Type Conversion1/1 -> MinMax/2
  Data Type Conversion4/1 -> MinMax1/1
  MinMax1/1 -> Data Type Conversion3/1
  LowerLimit/1 -> Data Type Conversion4/1
  MinMax/1 -> MinMax1/2
  IN/1 -> Data Type Conversion2/1
  UpperLimit/1 -> Data Type Conversion1/1

== system Kitchen_Lib/Kitchen/100ms/Kitchn/Subsystem1/Subsystem19/WaterTankEmptyDiagnostic/Diagno sticsDebouncing/DiagnosticsDebouncingOriginal/TurnOffDelayOriginal /TimePulseOriginal/RisingEdgeDetection ==
  CLK : Inport
  Constant : Constant  Value=boolean(1)  OutDataTypeStr=boolean
  Data Type Conversion1 : DataTypeConversion  OutDataTypeStr=boolean  SaturateOnIntegerOverflow=off  RndMeth=Floor
  Logical Operator : Logic  AllPortsSameDT=off  OutDataTypeStr=boolean
  Relational Operator : RelationalOperator  Operator=~=  OutDataTypeStr=boolean  InputSameDT=off
  Relational Operator1 : RelationalOperator  Operator===  OutDataTypeStr=boolean  InputSameDT=off
  Unit Delay : UnitDelay  SampleTime=-1  HasFrameUpgradeWarning=on
  Q : Outport
  wires:
  Data Type Conversion1/1 -> Relational Operator1/1, Relational Operator/2, Unit Delay/1
  Constant/1 -> Relational Operator1/2
  Logical Operator/1 -> Q/1
  Relational Operator1/1 -> Logical Operator/2
  Relational Operator/1 -> Logical Operator/1
  Unit Delay/1 -> Relational Operator/1
  CLK/1 -> Data Type Conversion1/1

== system Kitchen_Lib/Kitchen/100ms/Kitchn/Subsystem1/Subsystem19/WaterTankEmptyDiagnostic/Diagno sticsDebouncing/DiagnosticsDebouncingOriginal/TurnOffDelayOriginal /TimePulseOriginal/RisingEdgeDetection1 ==
  CLK : Inport
  Constant : Constant  Value=boolean(1)  OutDataTypeStr=boolean
  Data Type Conversion1 : DataTypeConversion  OutDataTypeStr=boolean  SaturateOnIntegerOverflow=off  RndMeth=Floor
  Logical Operator : Logic  AllPortsSameDT=off  OutDataTypeStr=boolean
  Relational Operator : RelationalOperator  Operator=~=  OutDataTypeStr=boolean  InputSameDT=off
  Relational Operator1 : RelationalOperator  Operator===  OutDataTypeStr=boolean  InputSameDT=off
  Unit Delay : UnitDelay  SampleTime=-1  HasFrameUpgradeWarning=on
  Q : Outport
  wires:
  Data Type Conversion1/1 -> Relational Operator1/1, Relational Operator/2, Unit Delay/1
  Constant/1 -> Relational Operator1/2
  Logical Operator/1 -> Q/1
  Relational Operator1/1 -> Logical Operator/2
  Relational Operator/1 -> Logical Operator/1
  Unit Delay/1 -> Relational Operator/1
  CLK/1 -> Data Type Conversion1/1

== system Kitchen_Lib/Kitchen/100ms/Kitchn/Subsystem1/Subsystem19/WaterTankEmptyDiagnostic/Diagno sticsDebouncing/DiagnosticsDebouncingOriginal/TurnOffDelayOriginal /TimePulseOriginal/SR ==
  S : Inport
  R : Inport  Port=2
  Constant1 : Constant  Value=boolean(1)  OutDataTypeStr=boolean
  Constant3 : Constant  Value=boolean(0)  OutDataTypeStr=boolean
  Data Type Conversion1 : DataTypeConversion  OutDataTypeStr=boolean  SaturateOnIntegerOverflow=off  RndMeth=Floor
  Data Type Conversion2 : DataTypeConversion  OutDataTypeStr=boolean  SaturateOnIntegerOverflow=off  RndMeth=Floor
  Multiport Switch : MultiPortSwitch  DataPortOrder=Zero-based contiguous  Inputs=2  zeroidx=on  SaturateOnIntegerOverflow=off  InputSameDT=off
  Multiport Switch1 : MultiPortSwitch  DataPortOrder=Zero-based contiguous  Inputs=2  zeroidx=on  SaturateOnIntegerOverflow=off  InputSameDT=off
  Unit Delay : UnitDelay  SampleTime=-1  HasFrameUpgradeWarning=on
  Q : Outport
  wires:
  Data Type Conversion2/1 -> Multiport Switch/1
  Data Type Conversion1/1 -> Multiport Switch1/1
  Constant3/1 -> Multiport Switch1/3
  Multiport Switch/1 -> Unit Delay/1, Q/1
  Unit Delay/1 -> Multiport Switch1/2
  R/1 -> Data Type Conversion1/1
  Multiport Switch1/1 -> Multiport Switch/2
  Constant1/1 -> Multiport Switch/3
  S/1 -> Data Type Conversion2/1

== system Kitchen_Lib/Kitchen/100ms/Kitchn/Subsystem1/Subsystem19/WaterTankEmptyDiagnostic/Diagno sticsDebouncing/DiagnosticsDebouncingOriginal/TurnOffDelayOriginal /TimePulseOriginal/TimerCountingUpOriginal ==
  TimerEnable : Inport
  TimerReset : Inport  Port=2
  TimerThreshold : Inport  Port=3
  CycleTime : Inport  Port=4
  Data Type Conversion2 : DataTypeConversion  OutDataTypeStr=boolean  SaturateOnIntegerOverflow=off  RndMeth=Floor
  Data Type Conversion4 : DataTypeConversion  OutDataTypeStr=uint32  SaturateOnIntegerOverflow=off  RndMeth=Floor
  Data Type Conversion5 : DataTypeConversion  OutDataTypeStr=uint32  SaturateOnIntegerOverflow=off  RndMeth=Floor
  Data Type Conversion6 : DataTypeConversion  OutDataTypeStr=uint32  SaturateOnIntegerOverflow=off  RndMeth=Floor
  Data Type Conversion7 : DataTypeConversion  OutDataTypeStr=boolean  SaturateOnIntegerOverflow=off  RndMeth=Floor
  Delay : Delay  DelayLength=1  InitialCondition=0  ExternalReset=Rising
      settings: InputPortMap=u0,r5
  Delay1 : Delay  DelayLength=1  InitialCondition=0
  Logical Operator1 : Logic  Operator=NOT  AllPortsSameDT=off  OutDataTypeStr=boolean
  Logical Operator2 : Logic  AllPortsSameDT=off  OutDataTypeStr=boolean
  Logical Operator3 : Logic  Operator=OR  AllPortsSameDT=off  OutDataTypeStr=boolean
  Multiport Switch : MultiPortSwitch  DataPortOrder=Zero-based contiguous  Inputs=2  zeroidx=on  SaturateOnIntegerOverflow=off  InputSameDT=off
  Multiport Switch1 : MultiPortSwitch  DataPortOrder=Zero-based contiguous  Inputs=2  zeroidx=on  SaturateOnIntegerOverflow=off  InputSameDT=off
  Multiport Switch2 : MultiPortSwitch  DataPortOrder=Zero-based contiguous  Inputs=2  zeroidx=on  SaturateOnIntegerOverflow=off  InputSameDT=off
  Relational Operator : RelationalOperator  OutDataTypeStr=boolean  InputSameDT=off
  Relational Operator1 : RelationalOperator  Operator===  OutDataTypeStr=boolean  InputSameDT=off
  RisingEdgeDetection : Subsystem  AncestorBlock=MAN_Library/RisingEdgeDetection
  StartValue_ms1 : Constant  Value=uint32(4294967295)  OutDataTypeStr=uint32
  StartValue_ms2 : Constant  Value=uint32(4294967295)  OutDataTypeStr=uint32
  StartValue_ms3 : Constant  Value=uint32(0)  OutDataTypeStr=uint32
  StartValue_ms5 : Constant  Value=uint32(4294967295)  OutDataTypeStr=uint32
  Sum : Sum
  U32_Saturation : Subsystem  AncestorBlock=MAN_Library/U32_Saturation
  TimerFlag : Outport
  TimerCurrentValue : Outport  Port=2
  wires:
  CycleTime/1 -> Data Type Conversion4/1
  Data Type Conversion2/1 -> Logical Operator3/1
  RisingEdgeDetection/1(Q) -> Logical Operator3/2
  TimerReset/1 -> Data Type Conversion2/1
  TimerEnable/1 -> Data Type Conversion7/1
  Data Type Conversion6/1 -> Relational Operator/2
  Data Type Conversion4/1 -> Sum/2
  StartValue_ms3/1 -> U32_Saturation/3(LowerLimit), Multiport Switch/3
  Multiport Switch2/1 -> U32_Saturation/2(IN)
  Sum/1 -> Multiport Switch2/2
  StartValue_ms2/1 -> Multiport Switch2/3
  Relational Operator1/1 -> Multiport Switch2/1
  Delay/1 -> Multiport Switch1/2, Relational Operator1/1, Sum/1
  StartValue_ms5/1 -> Relational Operator1/2
  Logical Operator3/1 -> Multiport Switch/1, [ResetTimer_BOOL]
  StartValue_ms1/1 -> U32_Saturation/1(UpperLimit)
  Delay1/1 -> Logical Operator1/1
  U32_Saturation/1(OUT) -> Multiport Switch1/3
  Logical Operator1/1 -> Logical Operator2/2
  Logical Operator2/1 -> Multiport Switch1/1
  Data Type Conversion5/1 -> TimerCurrentValue/1, Delay/1, Relational Operator/1
  Data Type Conversion7/1 -> Logical Operator2/1, RisingEdgeDetection/1(CLK)
  Multiport Switch/1 -> Data Type Conversion5/1
  Relational Operator/1 -> TimerFlag/1, Delay1/1
  Multiport Switch1/1 -> Multiport Switch/2
  TimerThreshold/1 -> Data Type Conversion6/1
  [ResetTimer_BOOL] -> Delay/2

== system Kitchen_Lib/Kitchen/100ms/Kitchn/Subsystem1/Subsystem19/WaterTankEmptyDiagnostic/Diagno sticsDebouncing/DiagnosticsDebouncingOriginal/TurnOnDelayOriginal/TimePulseOriginal/RisingEdgeDetection ==
  CLK : Inport
  Constant : Constant  Value=boolean(1)  OutDataTypeStr=boolean
  Data Type Conversion1 : DataTypeConversion  OutDataTypeStr=boolean  SaturateOnIntegerOverflow=off  RndMeth=Floor
  Logical Operator : Logic  AllPortsSameDT=off  OutDataTypeStr=boolean
  Relational Operator : RelationalOperator  Operator=~=  OutDataTypeStr=boolean  InputSameDT=off
  Relational Operator1 : RelationalOperator  Operator===  OutDataTypeStr=boolean  InputSameDT=off
  Unit Delay : UnitDelay  SampleTime=-1  HasFrameUpgradeWarning=on
  Q : Outport
  wires:
  Data Type Conversion1/1 -> Relational Operator1/1, Relational Operator/2, Unit Delay/1
  Constant/1 -> Relational Operator1/2
  Logical Operator/1 -> Q/1
  Relational Operator1/1 -> Logical Operator/2
  Relational Operator/1 -> Logical Operator/1
  Unit Delay/1 -> Relational Operator/1
  CLK/1 -> Data Type Conversion1/1

== system Kitchen_Lib/Kitchen/100ms/Kitchn/Subsystem1/Subsystem19/WaterTankEmptyDiagnostic/Diagno sticsDebouncing/DiagnosticsDebouncingOriginal/TurnOnDelayOriginal/TimePulseOriginal/RisingEdgeDetection1 ==
  CLK : Inport
  Constant : Constant  Value=boolean(1)  OutDataTypeStr=boolean
  Data Type Conversion1 : DataTypeConversion  OutDataTypeStr=boolean  SaturateOnIntegerOverflow=off  RndMeth=Floor
  Logical Operator : Logic  AllPortsSameDT=off  OutDataTypeStr=boolean
  Relational Operator : RelationalOperator  Operator=~=  OutDataTypeStr=boolean  InputSameDT=off
  Relational Operator1 : RelationalOperator  Operator===  OutDataTypeStr=boolean  InputSameDT=off
  Unit Delay : UnitDelay  SampleTime=-1  HasFrameUpgradeWarning=on
  Q : Outport
  wires:
  Data Type Conversion1/1 -> Relational Operator1/1, Relational Operator/2, Unit Delay/1
  Constant/1 -> Relational Operator1/2
  Logical Operator/1 -> Q/1
  Relational Operator1/1 -> Logical Operator/2
  Relational Operator/1 -> Logical Operator/1
  Unit Delay/1 -> Relational Operator/1
  CLK/1 -> Data Type Conversion1/1

== system Kitchen_Lib/Kitchen/100ms/Kitchn/Subsystem1/Subsystem19/WaterTankEmptyDiagnostic/Diagno sticsDebouncing/DiagnosticsDebouncingOriginal/TurnOnDelayOriginal/TimePulseOriginal/SR ==
  S : Inport
  R : Inport  Port=2
  Constant1 : Constant  Value=boolean(1)  OutDataTypeStr=boolean
  Constant3 : Constant  Value=boolean(0)  OutDataTypeStr=boolean
  Data Type Conversion1 : DataTypeConversion  OutDataTypeStr=boolean  SaturateOnIntegerOverflow=off  RndMeth=Floor
  Data Type Conversion2 : DataTypeConversion  OutDataTypeStr=boolean  SaturateOnIntegerOverflow=off  RndMeth=Floor
  Multiport Switch : MultiPortSwitch  DataPortOrder=Zero-based contiguous  Inputs=2  zeroidx=on  SaturateOnIntegerOverflow=off  InputSameDT=off
  Multiport Switch1 : MultiPortSwitch  DataPortOrder=Zero-based contiguous  Inputs=2  zeroidx=on  SaturateOnIntegerOverflow=off  InputSameDT=off
  Unit Delay : UnitDelay  SampleTime=-1  HasFrameUpgradeWarning=on
  Q : Outport
  wires:
  Data Type Conversion2/1 -> Multiport Switch/1
  Data Type Conversion1/1 -> Multiport Switch1/1
  Constant3/1 -> Multiport Switch1/3
  Multiport Switch/1 -> Unit Delay/1, Q/1
  Unit Delay/1 -> Multiport Switch1/2
  R/1 -> Data Type Conversion1/1
  Multiport Switch1/1 -> Multiport Switch/2
  Constant1/1 -> Multiport Switch/3
  S/1 -> Data Type Conversion2/1

== system Kitchen_Lib/Kitchen/100ms/Kitchn/Subsystem1/Subsystem19/WaterTankEmptyDiagnostic/Diagno sticsDebouncing/DiagnosticsDebouncingOriginal/TurnOnDelayOriginal/TimePulseOriginal/TimerCountingUpOriginal ==
  TimerEnable : Inport
  TimerReset : Inport  Port=2
  TimerThreshold : Inport  Port=3
  CycleTime : Inport  Port=4
  Data Type Conversion2 : DataTypeConversion  OutDataTypeStr=boolean  SaturateOnIntegerOverflow=off  RndMeth=Floor
  Data Type Conversion4 : DataTypeConversion  OutDataTypeStr=uint32  SaturateOnIntegerOverflow=off  RndMeth=Floor
  Data Type Conversion5 : DataTypeConversion  OutDataTypeStr=uint32  SaturateOnIntegerOverflow=off  RndMeth=Floor
  Data Type Conversion6 : DataTypeConversion  OutDataTypeStr=uint32  SaturateOnIntegerOverflow=off  RndMeth=Floor
  Data Type Conversion7 : DataTypeConversion  OutDataTypeStr=boolean  SaturateOnIntegerOverflow=off  RndMeth=Floor
  Delay : Delay  DelayLength=1  InitialCondition=0  ExternalReset=Rising
      settings: InputPortMap=u0,r5
  Delay1 : Delay  DelayLength=1  InitialCondition=0
  Logical Operator1 : Logic  Operator=NOT  AllPortsSameDT=off  OutDataTypeStr=boolean
  Logical Operator2 : Logic  AllPortsSameDT=off  OutDataTypeStr=boolean
  Logical Operator3 : Logic  Operator=OR  AllPortsSameDT=off  OutDataTypeStr=boolean
  Multiport Switch : MultiPortSwitch  DataPortOrder=Zero-based contiguous  Inputs=2  zeroidx=on  SaturateOnIntegerOverflow=off  InputSameDT=off
  Multiport Switch1 : MultiPortSwitch  DataPortOrder=Zero-based contiguous  Inputs=2  zeroidx=on  SaturateOnIntegerOverflow=off  InputSameDT=off
  Multiport Switch2 : MultiPortSwitch  DataPortOrder=Zero-based contiguous  Inputs=2  zeroidx=on  SaturateOnIntegerOverflow=off  InputSameDT=off
  Relational Operator : RelationalOperator  OutDataTypeStr=boolean  InputSameDT=off
  Relational Operator1 : RelationalOperator  Operator===  OutDataTypeStr=boolean  InputSameDT=off
  RisingEdgeDetection : Subsystem  AncestorBlock=MAN_Library/RisingEdgeDetection
  StartValue_ms1 : Constant  Value=uint32(4294967295)  OutDataTypeStr=uint32
  StartValue_ms2 : Constant  Value=uint32(4294967295)  OutDataTypeStr=uint32
  StartValue_ms3 : Constant  Value=uint32(0)  OutDataTypeStr=uint32
  StartValue_ms5 : Constant  Value=uint32(4294967295)  OutDataTypeStr=uint32
  Sum : Sum
  U32_Saturation : Subsystem  AncestorBlock=MAN_Library/U32_Saturation
  TimerFlag : Outport
  TimerCurrentValue : Outport  Port=2
  wires:
  CycleTime/1 -> Data Type Conversion4/1
  Data Type Conversion2/1 -> Logical Operator3/1
  RisingEdgeDetection/1(Q) -> Logical Operator3/2
  TimerReset/1 -> Data Type Conversion2/1
  TimerEnable/1 -> Data Type Conversion7/1
  Data Type Conversion6/1 -> Relational Operator/2
  Data Type Conversion4/1 -> Sum/2
  StartValue_ms3/1 -> U32_Saturation/3(LowerLimit), Multiport Switch/3
  Multiport Switch2/1 -> U32_Saturation/2(IN)
  Sum/1 -> Multiport Switch2/2
  StartValue_ms2/1 -> Multiport Switch2/3
  Relational Operator1/1 -> Multiport Switch2/1
  Delay/1 -> Multiport Switch1/2, Relational Operator1/1, Sum/1
  StartValue_ms5/1 -> Relational Operator1/2
  Logical Operator3/1 -> Multiport Switch/1, [ResetTimer_BOOL]
  StartValue_ms1/1 -> U32_Saturation/1(UpperLimit)
  Delay1/1 -> Logical Operator1/1
  U32_Saturation/1(OUT) -> Multiport Switch1/3
  Logical Operator1/1 -> Logical Operator2/2
  Logical Operator2/1 -> Multiport Switch1/1
  Data Type Conversion5/1 -> TimerCurrentValue/1, Delay/1, Relational Operator/1
  Data Type Conversion7/1 -> Logical Operator2/1, RisingEdgeDetection/1(CLK)
  Multiport Switch/1 -> Data Type Conversion5/1
  Relational Operator/1 -> TimerFlag/1, Delay1/1
  Multiport Switch1/1 -> Multiport Switch/2
  TimerThreshold/1 -> Data Type Conversion6/1
  [ResetTimer_BOOL] -> Delay/2

== system Kitchen_Lib/Kitchen/100ms/Kitchn/Subsystem1/Subsystem19/WaterTankEmptyDiagnostic/TurnOffDelay/TurnOffDelayOriginal/TimePulseOriginal/TimerCountingUpOriginal/RisingEdgeDetection ==
  CLK : Inport
  Constant : Constant  Value=boolean(1)  OutDataTypeStr=boolean
  Data Type Conversion1 : DataTypeConversion  OutDataTypeStr=boolean  SaturateOnIntegerOverflow=off  RndMeth=Floor
  Logical Operator : Logic  AllPortsSameDT=off  OutDataTypeStr=boolean
  Relational Operator : RelationalOperator  Operator=~=  OutDataTypeStr=boolean  InputSameDT=off
  Relational Operator1 : RelationalOperator  Operator===  OutDataTypeStr=boolean  InputSameDT=off
  Unit Delay : UnitDelay  SampleTime=-1  HasFrameUpgradeWarning=on
  Q : Outport
  wires:
  Data Type Conversion1/1 -> Relational Operator1/1, Relational Operator/2, Unit Delay/1
  Constant/1 -> Relational Operator1/2
  Logical Operator/1 -> Q/1
  Relational Operator1/1 -> Logical Operator/2
  Relational Operator/1 -> Logical Operator/1
  Unit Delay/1 -> Relational Operator/1
  CLK/1 -> Data Type Conversion1/1

== system Kitchen_Lib/Kitchen/100ms/Kitchn/Subsystem1/Subsystem19/WaterTankEmptyDiagnostic/TurnOffDelay/TurnOffDelayOriginal/TimePulseOriginal/TimerCountingUpOriginal/U32_Saturation ==
  UpperLimit : Inport
  IN : Inport  Port=2
  LowerLimit : Inport  Port=3
  Data Type Conversion{1..4} (4 alike) : DataTypeConversion  OutDataTypeStr=uint32  SaturateOnIntegerOverflow=off  RndMeth=Floor
  MinMax : MinMax  Inputs=2  OutDataTypeStr=uint32
  MinMax1 : MinMax  Function=max  Inputs=2  OutDataTypeStr=uint32
  OUT : Outport
  wires:
  Data Type Conversion3/1 -> OUT/1
  Data Type Conversion2/1 -> MinMax/1
  Data Type Conversion1/1 -> MinMax/2
  Data Type Conversion4/1 -> MinMax1/1
  MinMax1/1 -> Data Type Conversion3/1
  LowerLimit/1 -> Data Type Conversion4/1
  MinMax/1 -> MinMax1/2
  IN/1 -> Data Type Conversion2/1
  UpperLimit/1 -> Data Type Conversion1/1

== system Kitchen_Lib/Kitchen/100ms/Kitchn/Subsystem1/Subsystem16/001_KitchnCtl/002_FlipFlop/KitchenEnable/Subsystem/TurnOnDelay/TurnOnDelayOriginal/RisingEdgeDetection ==
  CLK : Inport
  Constant : Constant  Value=boolean(1)  OutDataTypeStr=boolean
  Data Type Conversion1 : DataTypeConversion  OutDataTypeStr=boolean  SaturateOnIntegerOverflow=off  RndMeth=Floor
  Logical Operator : Logic  AllPortsSameDT=off  OutDataTypeStr=boolean
  Relational Operator : RelationalOperator  Operator=~=  OutDataTypeStr=boolean  InputSameDT=off
  Relational Operator1 : RelationalOperator  Operator===  OutDataTypeStr=boolean  InputSameDT=off
  Unit Delay : UnitDelay  SampleTime=-1  HasFrameUpgradeWarning=on
  Q : Outport
  wires:
  Data Type Conversion1/1 -> Relational Operator1/1, Relational Operator/2, Unit Delay/1
  Constant/1 -> Relational Operator1/2
  Logical Operator/1 -> Q/1
  Relational Operator1/1 -> Logical Operator/2
  Relational Operator/1 -> Logical Operator/1
  Unit Delay/1 -> Relational Operator/1
  CLK/1 -> Data Type Conversion1/1
